simulink model "final"  (R2019b)
settings: Solver=VariableStepAuto  StartTime=0.0  StopTime=5e-2  RelTol=1e-3
values from neighbouring files (symbols this model uses):
  filter = rcosdesign(alpha,symNum,sym,'sqrt')    [loopFil.m]
undefined symbols (not defined in the file or in its folder): ag, bg, Gg
libraries: dspsigops x6, dspsrcs4 x1
settings Model: Creator=Administrator  LastModifiedBy=Administrator

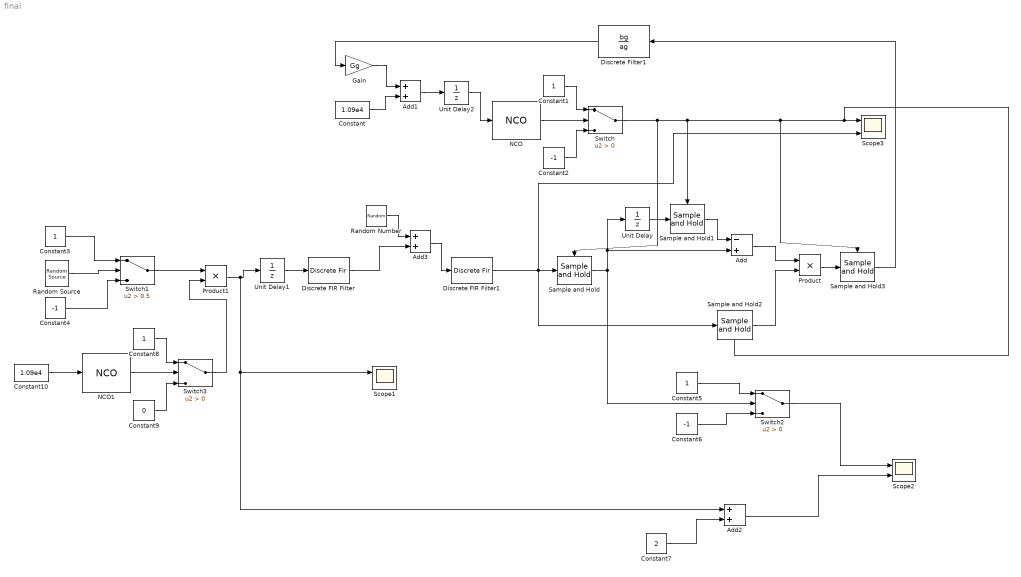
== system final ==
  Add : Sum  Inputs=-+
  Add1 : Sum  OutDataTypeStr=int16
  Add2 : Sum  OutDataTypeStr=int16
  Add3 : Sum  OutDataTypeStr=int16
  Constant : Constant  Value=1.09e4  OutDataTypeStr=int32  SampleTime=1/(6*19.2e3)
  Constant{1,3,5,8} (4 alike) : Constant  SampleTime=1/(6*19.2e3)
  Constant10 : Constant  Value=1.09e4  OutDataTypeStr=int32  SampleTime=1/(6*19.2e3)
  Constant2 : Constant  Value=-1  SampleTime=1/(6*19.2e3)
  Constant4 : Constant  Value=-1  SampleTime=1/(6*19.2e3)
  Constant6 : Constant  Value=-1  SampleTime=1/(6*19.2e3)
  Constant7 : Constant  Value=2  SampleTime=1/(6*19.2e3)
  Constant9 : Constant  Value=0  SampleTime=1/(6*19.2e3)
  Discrete FIR Filter : DiscreteFir  Coefficients=filter
  Discrete FIR Filter1 : DiscreteFir  Coefficients=filter
  Discrete Filter1 : DiscreteFilter  Numerator=bg  Denominator=ag
  Gain : Gain  Gain=Gg  OutDataTypeStr=int32
  NCO : dspsigops/NCO  AccIncSrc=Input port  AccInc=100  PhaseOffsetSrc=Specify via dialog  PhaseOffset=0  AccumWL=16  HasDither=on  DitherWL=4  PNgeneratorLength=19  HasPhaseQuantizer=on  TableDepth=12  HasOutputPhaseError=off  Formula=Sine  DataType=single  OutputWL=16  OutputFL=14  CompMethod=Table lookup (no interpolation)  SampleTime=1  SamplesPerFrame=1  OutputFrames=off
      settings: SourceProductName=DSP System Toolbox  SourceProductBaseCode=DS
  NCO1 : dspsigops/NCO  AccIncSrc=Input port  AccInc=100  PhaseOffsetSrc=Specify via dialog  PhaseOffset=0  AccumWL=16  HasDither=on  DitherWL=4  PNgeneratorLength=19  HasPhaseQuantizer=on  TableDepth=12  HasOutputPhaseError=off  Formula=Sine  DataType=single  OutputWL=16  OutputFL=14  CompMethod=Table lookup (no interpolation)  SampleTime=1  SamplesPerFrame=1  OutputFrames=off
      settings: SourceProductName=DSP System Toolbox  SourceProductBaseCode=DS
  Product : Product
  Product1 : Product
  Random Number : RandomNumber  Variance=0.01  SampleTime=1/(6*19.2e3)
  Random Source : dspsrcs4/Random Source  SrcType=Uniform  NormMethod=Ziggurat  CltLength=12  MinVal=0  MaxVal=1  MeanVal=0  VarVal=1  RepMode=Not repeatable  rawSeed=1  IsInherit=off  SampMode=Discrete  SampTime=1/(19.2e3)  SampFrame=1  DataType=Double  OutComplex=Real  OutputFrames=off
  Sample and Hold : dspsigops/Sample and Hold  trig=Rising edge  initCond=0  latchinput=off
  Sample and Hold1 : dspsigops/Sample and Hold  trig=Rising edge  initCond=0  latchinput=off
  Sample and Hold2 : dspsigops/Sample and Hold  trig=Falling edge  initCond=0  latchinput=off
  Sample and Hold3 : dspsigops/Sample and Hold  Tag=error  trig=Rising edge  initCond=0  latchinput=off
  Scope1 : Scope  NumInputPorts=2
  Scope2 : Scope  NumInputPorts=2
  Scope3 : Scope  NumInputPorts=3
  Switch : Switch  Criteria=u2 > Threshold
  Switch1 : Switch  Criteria=u2 > Threshold  Threshold=0.5
  Switch2 : Switch  Criteria=u2 > Threshold
  Switch3 : Switch  Criteria=u2 > Threshold
  Unit Delay : UnitDelay  SampleTime=-1  HasFrameUpgradeWarning=on
  Unit Delay1 : UnitDelay  SampleTime=-1  HasFrameUpgradeWarning=on
  Unit Delay2 : UnitDelay  SampleTime=-1  HasFrameUpgradeWarning=on
  wires:
  Switch/1 -> Sample and Hold1/Trigger, Scope3/1, Sample and Hold2/Trigger, Sample and Hold3/Trigger, Sample and Hold/Trigger
  Sample and Hold3/1 -> Discrete Filter1/1
  Product/1 -> Sample and Hold3/1
  Add/1 -> Product/1
  Sample and Hold2/1 -> Product/2
  Sample and Hold1/1 -> Add/1
  Unit Delay/1 -> Sample and Hold1/1
  Sample and Hold/1 -> Unit Delay/1, Add/2, Switch2/2
  Discrete FIR Filter1/1 -> Sample and Hold/1, Scope3/3, Sample and Hold2/1
  Constant1/1 -> Switch/1
  NCO/1 -> Switch/2
  Unit Delay2/1 -> NCO/1
  Constant/1 -> Add1/2
  Add1/1 -> Unit Delay2/1
  Gain/1 -> Add1/1
  Constant2/1 -> Switch/3
  Random Source/1 -> Switch1/2
  Unit Delay1/1 -> Discrete FIR Filter/1
  Constant3/1 -> Switch1/1
  Constant4/1 -> Switch1/3
  Constant6/1 -> Switch2/3
  Constant5/1 -> Switch2/1
  Switch2/1 -> Scope2/1
  Constant7/1 -> Add2/2
  Add2/1 -> Scope2/2
  Constant8/1 -> Switch3/1
  Constant9/1 -> Switch3/3
  NCO1/1 -> Switch3/2
  Constant10/1 -> NCO1/1
  Switch1/1 -> Product1/1
  Product1/1 -> Add2/1, Scope1/1, Unit Delay1/1
  Discrete FIR Filter/1 -> Add3/2
  Random Number/1 -> Add3/1
  Add3/1 -> Discrete FIR Filter1/1
  Switch3/1 -> Product1/2
  Discrete Filter1/1 -> Gain/1
